simulink model "quadrotor_linear_obsv_model_submission"  (R2019a)
settings: Solver=VariableStepAuto  StartTime=0.0  StopTime=10.0  RelTol=1e-3
undefined symbols (not defined in the file): C, g, K, L, m, nl_update, x0, xhat0
settings Model: Creator=tmcnama2  LastModifiedBy=tmcnama2
settings DataIOCC: InitialState=x0
settings DebuggingCC: InitInArrayFormatMsg=none

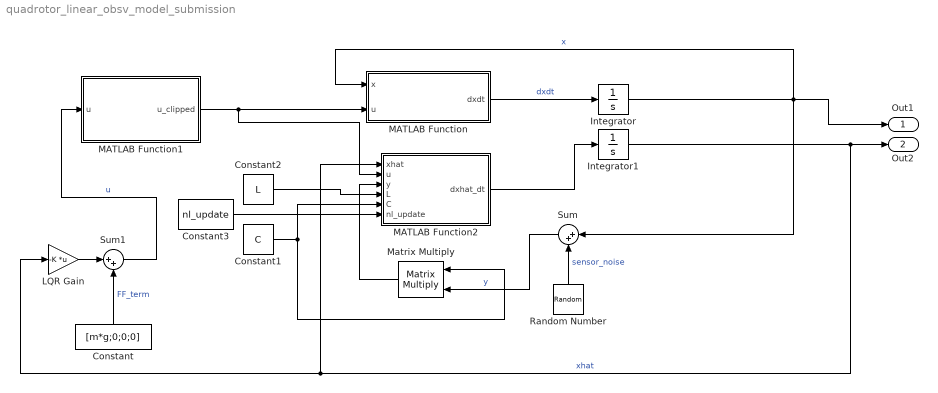
== system quadrotor_linear_obsv_model_submission ==
  Constant : Constant  Value=[m*g;0;0;0]  VectorParams1D=off
  Constant1 : Constant  Value=C
  Constant2 : Constant  Value=L
  Constant3 : Constant  Value=nl_update
  Integrator : Integrator  InitialCondition=x0
  Integrator1 : Integrator  InitialCondition=xhat0
  "LQR Gain " : Gain  Gain=-K  Multiplication=Matrix(K*u)
  MATLAB Function : MATLAB Function  TreatAsAtomicUnit=on
  MATLAB Function1 : MATLAB Function  TreatAsAtomicUnit=on
  MATLAB Function2 : MATLAB Function  TreatAsAtomicUnit=on
  Matrix Multiply : Product  Multiplication=Matrix(*)
  Random Number : RandomNumber  Mean=zeros(12,1)  Variance=.0001*ones(12,1)  SampleTime=0.1  VectorParams1D=off
  Sum : Sum  Inputs=|++
  Sum1 : Sum  Inputs=|++
  Out1 : Outport  SignalName=x
  Out2 : Outport  Port=2  SignalName=xhat
  wires:
  Random Number/1 -> Sum/2  "sensor_noise"
  Constant/1 -> Sum1/2  "FF_term"
  "LQR Gain "/1 -> Sum1/1
  Sum1/1 -> MATLAB Function1/1(u)  "u"
  MATLAB Function2/1(dxhat_dt) -> Integrator1/1
  MATLAB Function1/1(u_clipped) -> MATLAB Function2/2(u), MATLAB Function/2(u)
  MATLAB Function/1(dxdt) -> Integrator/1  "dxdt"
  Integrator/1 -> MATLAB Function/1(x), Sum/1, Out1/1  "x"
  Integrator1/1 -> MATLAB Function2/1(xhat), "LQR Gain "/1, Out2/1  "xhat"
  Constant1/1 -> Matrix Multiply/1, MATLAB Function2/5(C)
  Constant2/1 -> MATLAB Function2/4(L)
  Matrix Multiply/1 -> MATLAB Function2/3(y)
  Sum/1 -> Matrix Multiply/2  "y"
  Constant3/1 -> MATLAB Function2/6(nl_update)

== matlab function quadrotor_linear_obsv_model_submission/MATLAB Function1 ==
  data: u input; u_clipped output
function u_clipped = input_norm(u)
u_clipped = zeros(4,1);
u_clipped(1) = max([min([u(1), 16]),0]);
u_clipped(2) = max([min([u(2), .432]),-.432]);
u_clipped(3) = max([min([u(3), .432]),-.432]);
u_clipped(4) = max([min([u(4), .1]),-.1]);

== matlab function quadrotor_linear_obsv_model_submission/MATLAB Function ==
  data: x input; u input; dxdt output
function dxdt = quadrotor_dynamics(x, u)
    m = 0.6;
    Jx = 0.0092;
    Jy = 0.0091;
    Jz = 0.0101;
    g = 9.81;
    px_dot = x(1);
%   px =     x(2);
    py_dot = x(3);
%   py =     x(4);
    pz_dot = x(5);
%   pz =     x(6);
    p =      x(7);
    phi =    x(8);
    q =      x(9); 
    theta =  x(10);
    r =      x(11);
    psi =    x(12);
    
    u_clipped = u;
    
    F = u_clipped(1);
    tau_phi = u_clipped(2);
    tau_theta = u_clipped(3);
    tau_psi = u_clipped(4);
    
    az = -F/m;
    dxdt = zeros(12,1);
    dxdt =  [cos(phi)*sin(theta)*az;
             px_dot;
             -sin(phi)*az;
             py_dot;
             g + cos(phi)*cos(theta)*az;
             pz_dot;             
             1/Jx*tau_phi;
             p + q*sin(phi)*tan(theta) + r*cos(phi)*tan(theta);
             1/Jy*tau_theta;
             q*cos(phi) - r*sin(phi);
             1/Jz*tau_psi;
             q*sin(phi)/cos(theta) + r*cos(phi)/cos(theta)];

== matlab function quadrotor_linear_obsv_model_submission/MATLAB Function2 ==
  data: xhat input; u input; dxhat_dt output; y input; L input; C input; nl_update input
function dxhat_dt = observer_dynamics(xhat, u, y, L, C, nl_update)
% dx_hat_dt = A*xhat + B*u + L*(y-xhat);
    A = [0         0         0         0         0         0         0         0         0   -9.8000         0         0;
    1.0000         0         0         0         0         0         0         0         0         0         0         0;
         0         0         0         0         0         0         0    9.8000         0         0         0         0;
         0         0    1.0000         0         0         0         0         0         0         0         0         0;
         0         0         0         0         0         0         0         0         0         0         0         0;
         0         0         0         0    1.0000         0         0         0         0         0         0         0;
         0         0         0         0         0         0         0         0         0         0         0         0;
         0         0         0         0         0         0    1.0000         0         0         0         0         0;
         0         0         0         0         0         0         0         0         0         0         0         0;
         0         0         0         0         0         0         0         0    1.0000         0         0         0;
         0         0         0         0         0         0         0         0         0         0         0         0;
         0         0         0         0         0         0         0         0         0         0    1.0000         0];
    B = [         0         0         0         0;
         0         0         0         0;
         0         0         0         0;
         0         0         0         0;
   -1.6667         0         0         0;
         0         0         0         0;
         0  108.6957         0         0;
         0         0         0         0;
         0         0  109.8901         0;
         0         0         0         0;
         0         0         0   99.0099;
         0         0         0         0];
    if ~nl_update    
        dxhat_dt = zeros(12,1);
        dxhat_dt(1:12) = A*xhat+B*u + L*(y-C*xhat);
    else
        m = 0.6;
        Jx = 0.0092;
        Jy = 0.0091;
        Jz = 0.0101;
        g = 9.81;
        px_dot = xhat(1);
    %   px =     x(2);
        py_dot = xhat(3);
    %   py =     x(4);
        pz_dot = xhat(5);
    %   pz =     x(6);
        p =      xhat(7);
        phi =    xhat(8);
        q =      xhat(9); 
        theta =  xhat(10);
        r =      xhat(11);
        psi =    xhat(12);

        u_clipped = u;

        F = u_clipped(1);
        tau_phi = u_clipped(2);
        tau_theta = u_clipped(3);
        tau_psi = u_clipped(4);

        az = -F/m;
        dxhat_dt = zeros(12,1);
        dxhat_dt(1) = cos(phi)*sin(theta)*az;
        dxhat_dt(2) = px_dot;
        dxhat_dt(3) = -sin(phi)*az;
        dxhat_dt(4) = py_dot;
        dxhat_dt(5) = g + cos(phi)*cos(theta)*az;
        dxhat_dt(6) = pz_dot;             
        dxhat_dt(7) = 1/Jx*tau_phi;
        dxhat_dt(8) = p + q*sin(phi)*tan(theta) + r*cos(phi)*tan(theta);
        dxhat_dt(9) = 1/Jy*tau_theta;
        dxhat_dt(10)=  q*cos(phi) - r*sin(phi);
        dxhat_dt(11)=  1/Jz*tau_psi;
        dxhat_dt(12)= q*sin(phi)/cos(theta) + r*cos(phi)/cos(theta);
        dxhat_dt = dxhat_dt + L*(y-C*xhat);
    end
